simulink model "immd_design_elen_sim2"  (R2013a)
settings: Solver=ode4  StartTime=0.0  StopTime=0.04  FixedStep=Ts  RelTol=1e-3
values from neighbouring files (symbols this model uses):
  Cdc = ma*(Iapeak - Idcc)/(volt_ripple*fsw*2)    [immd_design_elen.m]    (also in immd_efficiency.m = 5e-05; immd_simulation_base.m = 5e-05; sixth_harmonic_report.m = 0.003)
  Lload = Xload/wout_fund    [acemp_sixth.m]    (also in immd_base_varyingmod.m = Xload/wout; immd_design_elen.m = Xload/wout; immd_efficiency.m = Xload/wout; immd_simulation_base.m = Xload/wout)
  ma = 1    [IMMD_design_tool_v01.m]    (also in IMMD_design_tool_v02.m = 0.9; immd_base_varyingmod.m; immd_design_elen.m = 0.8; immd_efficiency.m = 0.85)
  phase = zeros(1,max_number_module)    [immd_base_varyingmod.m]    (also in immd_design_elen.m = [0 90 0 90]; immd_simulation_base.m = zeros(1,n))
  Rin = 10    [immd_design_elen.m]
  Rload = Zload*pf    [acemp_sixth.m]    (also in immd_base_varyingmod.m; immd_design_elen.m; immd_efficiency.m; immd_simulation_base.m)
  Ts = 1e-6    (= 1e-06)    [acemp_sixth.m]    (also in immd_base_varyingmod.m = 1e-05; immd_design_elen.m; immd_efficiency.m; immd_simulation_base.m)
  Vin = Vdc + Rin*(Ptotal/Vdc)    (= 704.609053498)    [immd_design_elen.m]
  wout = 2*pi*fout    (= 314.159265359)    [immd_base_varyingmod.m]    (also in immd_design_elen.m; immd_efficiency.m; immd_simulation_base.m)
undefined symbols (not defined in the file or in its folder): Lin
libraries: powerlib x65, powerlib_meascontrol x30
settings Model: Creator=ugurm  LastModifiedBy=ugurm

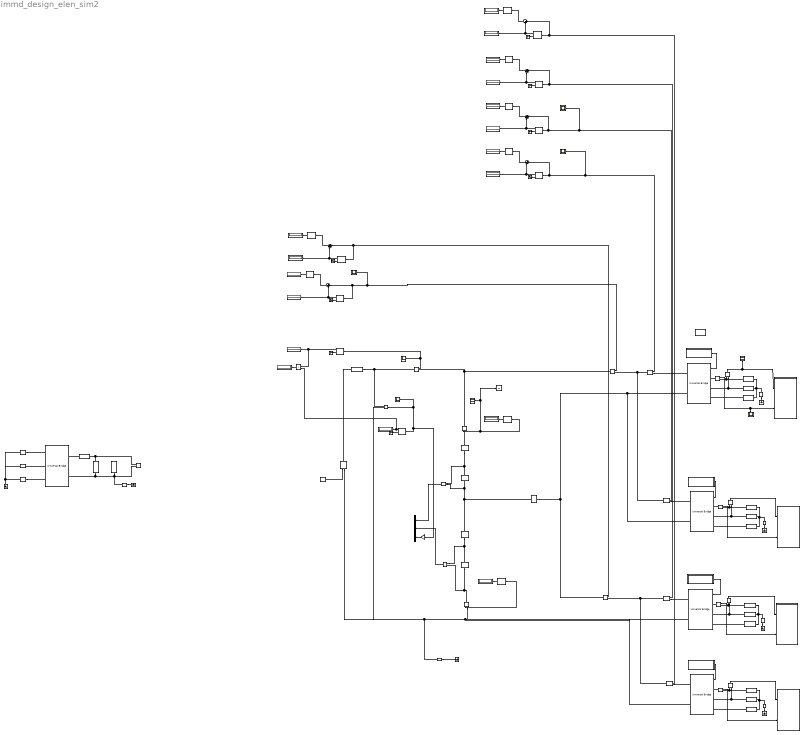
== system immd_design_elen_sim2 ==
  AC Voltage Source : powerlib/Electrical Sources/AC Voltage Source  Amplitude=230*sqrt(2)  Phase=0  Frequency=50  SampleTime=0  Measurements=None
  AC Voltage Source1 : powerlib/Electrical Sources/AC Voltage Source  Amplitude=230*sqrt(2)  Phase=120  Frequency=50  SampleTime=0  Measurements=None
  AC Voltage Source2 : powerlib/Electrical Sources/AC Voltage Source  Amplitude=230*sqrt(2)  Phase=240  Frequency=50  SampleTime=0  Measurements=None
  Constant : Constant  Value=Vin
  Display{1..10,15..21} (17 alike) : Display
  Fourier{1..8} (8 alike) : powerlib_meascontrol/Measurements/Fourier  Freq=fout  n=0  InInit=[20, 0]  Ts=Ts
  Gain : Gain  Gain=0.5
  Gate drive 1 : Subsystem
  Gate drive 2 : Subsystem
  Gate drive 3 : Subsystem
  Gate drive 4 : Subsystem
  Ground{,1..6} (7 alike) : powerlib/Elements/Ground  LConnTagsString=a
  Idc_m{1..13} (13 alike) : powerlib/Measurements/Current Measurement  PhasorSimulation=off  OutputType=Complex  PSBequivalent=0
  Integrator : Integrator
  Mux1 : Mux  Inputs=3
  Product : Product
  RMS1 : powerlib_meascontrol/Measurements/RMS  TrueRMS=on  Freq=50  RMSInit=0  Ts=Ts
  RMS{3..5,10..12} (6 alike) : powerlib_meascontrol/Measurements/RMS  TrueRMS=on  Freq=50  RMSInit=25  Ts=Ts
  RMS2 : powerlib_meascontrol/Measurements/RMS  TrueRMS=on  Freq=100  RMSInit=0  Ts=Ts
  Scope{4,9..10,12..16} (8 alike) : Scope
      Scope10 settings: YMin=-27.5  YMax=27.5  SaveName=ScopeData9
      Scope12 settings: YMin=-15  YMax=17.5  SaveName=Icap
      Scope13 settings: YMin=-15  YMax=17.5  SaveName=Idc1
      Scope14 settings: YMin=-9  SaveName=Iin
      Scope15 settings: YMin=-15  YMax=17.5  SaveName=Idc2
      Scope16 settings: YMin=-15  YMax=17.5  SaveName=Idct
      Scope4 settings: YMin=0  YMax=650  SaveName=Vdcc
      Scope9 settings: YMin=-25  YMax=425  SaveName=ScopeData8
  Series RLC Branch{,1..2,8..10,12..14,16..18} (12 alike) : powerlib/Elements/Series RLC Branch  LConnTagsString=__new0  RConnTagsString=__new0  BranchType=RL  Resistance=Rload  Inductance=Lload  SetiL0=off  InitialCurrent=0  Capacitance=1e-6  Setx0=off  InitialVoltage=0  Measurements=None
  Series RLC Branch{3..4,11,15,19,25} (6 alike) : powerlib/Elements/Series RLC Branch  LConnTagsString=__new0  RConnTagsString=__new0  BranchType=R  Resistance=1e12  Inductance=Lload  SetiL0=off  InitialCurrent=0  Capacitance=1e-6  Setx0=off  InitialVoltage=0  Measurements=None
  Series RLC Branch22 : powerlib/Elements/Series RLC Branch  LConnTagsString=__new0  RConnTagsString=__new0  BranchType=RL  Resistance=1e-3  Inductance=3e-3  SetiL0=off  InitialCurrent=0  Capacitance=1e-6  Setx0=off  InitialVoltage=0  Measurements=None
  Series RLC Branch23 : powerlib/Elements/Series RLC Branch  LConnTagsString=__new0  RConnTagsString=__new0  BranchType=RC  Resistance=1e-3  Inductance=3e-3  SetiL0=off  InitialCurrent=0  Capacitance=5e-3  Setx0=on  InitialVoltage=500  Measurements=None
  Series RLC Branch24 : powerlib/Elements/Series RLC Branch  LConnTagsString=__new0  RConnTagsString=__new0  BranchType=R  Resistance=36.45  Inductance=3e-3  SetiL0=off  InitialCurrent=0  Capacitance=1e-6  Setx0=off  InitialVoltage=0  Measurements=None
  Series RLC Branch26 : powerlib/Elements/Series RLC Branch  LConnTagsString=__new0  RConnTagsString=__new0  BranchType=R  Resistance=Rin  Inductance=Lin  SetiL0=off  InitialCurrent=0  Capacitance=1e-6  Setx0=off  InitialVoltage=0  Measurements=None
  Series RLC Branch27 : powerlib/Elements/Series RLC Branch  LConnTagsString=__new0  RConnTagsString=__new0  BranchType=C  Resistance=100e-6  Inductance=100e-6  SetiL0=off  InitialCurrent=0  Capacitance=Cdc*2  Setx0=off  InitialVoltage=170  Measurements=None
  Series RLC Branch28 : powerlib/Elements/Series RLC Branch  LConnTagsString=__new0  RConnTagsString=__new0  BranchType=R  Resistance=1e-9  Inductance=100e-6  SetiL0=off  InitialCurrent=0  Capacitance=Cdc*2  Setx0=on  InitialVoltage=170  Measurements=None
  Series RLC Branch29 : powerlib/Elements/Series RLC Branch  LConnTagsString=__new0  RConnTagsString=__new0  BranchType=R  Resistance=1e-9  Inductance=100e-6  SetiL0=off  InitialCurrent=0  Capacitance=Cdc*2  Setx0=on  InitialVoltage=170  Measurements=None
  Series RLC Branch30 : powerlib/Elements/Series RLC Branch  LConnTagsString=__new0  RConnTagsString=__new0  BranchType=R  Resistance=1e-9  Inductance=100e-6  SetiL0=off  InitialCurrent=0  Capacitance=Cdc*2  Setx0=on  InitialVoltage=170  Measurements=None
  Series RLC Branch5 : powerlib/Elements/Series RLC Branch  LConnTagsString=__new0  RConnTagsString=__new0  BranchType=C  Resistance=100e-6  Inductance=100e-6  SetiL0=off  InitialCurrent=0  Capacitance=Cdc*2  Setx0=off  InitialVoltage=170  Measurements=None
  Subsystem : Subsystem
  Subsystem1 : Subsystem
  Subsystem2 : Subsystem
  Subsystem3 : Subsystem
  Sum{1..6} (6 alike) : Sum  Inputs=|+-
  Terminator{1..8} (8 alike) : Terminator
  Universal Bridge{,1..3} (4 alike) : powerlib/Power Electronics/Universal Bridge  Arms=3  SnubberResistance=1e5  SnubberCapacitance=inf  Device=IGBT / Diodes  Ron=1e-6  Lon=0  ForwardVoltages="[  0  0  ]"  ForwardVoltage=0  GTOparameters=[ 10e-6 , 20e-6 ]  IGBTparameters=[0,0]  Measurements=None  Measurements_2=None  converterType=Rectifier
  Universal Bridge4 : powerlib/Power Electronics/Universal Bridge  Arms=3  SnubberResistance=1e5  SnubberCapacitance=inf  Device=Diodes  Ron=1e-6  Lon=0  ForwardVoltages="[  0  0  ]"  ForwardVoltage=0  GTOparameters=[ 10e-6 , 20e-6 ]  IGBTparameters=[0,0]  Measurements=None  Measurements_2=None  converterType=Rectifier
  Vdc : powerlib/Electrical Sources/Controlled Voltage Source  Initialize=off  Source_Type=DC  Amplitude=200  Phase=0  Frequency=0  Measurements=None
  Vdc_m{1..4} (4 alike) : powerlib/Measurements/Voltage Measurement  PhasorSimulation=off  OutputType=Complex  PSBequivalent=0
  Voltage Measurement{,1..3} (4 alike) : powerlib/Measurements/Voltage Measurement  PhasorSimulation=off  OutputType=Complex  PSBequivalent=0
  powergui : powerlib/powergui  Priority=1  SimulationMode=Discrete  SolverType=Tustin  SampleTime=Ts  frequency=60  SPID=off  DisableSnubberDevices=off  DisableRonSwitches=off  DisableVfSwitches=off  SwTol=0  Interpol=off  DisplayEquations=off  frequencyindice=0  Pbase=100e6  ErrMax=1e-4  Iterations=50  UnitsV=kV  UnitsW=MW  FunctionMessages=off  echomessages=off  HookPort=off  EnableUseOfTLC=off  x0status=blocks  RestoreLinks=warning  ResistiveCurrentMeasurement=off  Frange=[0:2:500]  Ylog=off  Xlog=on  ShowGrid=off  save=off  variable=ZData  structure=Vdc  ZoomFFT=off  StartTime=0.04  cycles=5  DisplayStyle=5  fundamental=50  FreqAxis=off  MaxFrequency=30000  frequencyindicesteady=1  RmsSteady=1  display=off  Ts=0  methode=off
  wires:
  Gate drive 1/1(gate1) -> Universal Bridge/1
  Vdc_m1/1 -> Scope9/1, Subsystem/1(Vab)
  Idc_m1/1 -> Scope10/1, Subsystem/2(Ia)
  Constant/1 -> Vdc/1
  RMS1/1 -> Display4/1
  Gate drive 2/1(gate1) -> Universal Bridge1/1
  Vdc_m2/1 -> Subsystem1/1(Vab)
  Idc_m2/1 -> Subsystem1/2(Ia)
  Gate drive 3/1(gate1) -> Universal Bridge2/1
  Vdc_m3/1 -> Subsystem2/1(Vab)
  Idc_m3/1 -> Subsystem2/2(Ia)
  Gate drive 4/1(gate1) -> Universal Bridge3/1
  Vdc_m4/1 -> Subsystem3/1(Vab)
  Idc_m4/1 -> Subsystem3/2(Ia)
  Product/1 -> Display3/1
  Fourier3/2 -> Terminator3/1
  Fourier3/1 -> Product/1, Display7/1
  Voltage Measurement1/1 -> Gain/1, Fourier4/1, Scope4/1
  Fourier4/2 -> Terminator5/1
  Fourier4/1 -> Product/2, Display9/1
  Idc_m7/1 -> Scope14/1, Fourier3/1
  RMS2/1 -> Display1/1
  RMS5/1 -> Display6/1
  Sum1/1 -> RMS5/1
  Fourier1/1 -> Sum1/2, Display5/1
  Fourier1/2 -> Terminator1/1
  Idc_m5/1 -> Scope16/1, Fourier1/1, Sum1/1
  RMS4/1 -> Display10/1
  Sum2/1 -> RMS4/1
  Fourier2/1 -> Sum2/2, Display2/1
  Fourier2/2 -> Terminator2/1
  Idc_m10/1 -> Fourier2/1, Sum2/1
  Idc_m11/1 -> Integrator/1, Scope12/1, RMS2/1
  Idc_m9/1 -> RMS1/1
  Voltage Measurement3/1 -> Mux1/2
  Voltage Measurement2/1 -> Mux1/1
  Idc_m8/1 -> Scope13/1, Sum3/1, Fourier5/1
  Idc_m13/1 -> Sum5/1, Fourier7/1
  Idc_m12/1 -> Sum6/1, Fourier8/1
  Idc_m6/1 -> Scope15/1, Sum4/1, Fourier6/1
  RMS3/1 -> Display8/1
  Sum3/1 -> RMS3/1
  Fourier5/1 -> Sum3/2, Display15/1
  Fourier5/2 -> Terminator4/1
  RMS10/1 -> Display16/1
  Sum4/1 -> RMS10/1
  Fourier6/1 -> Sum4/2, Display17/1
  Fourier6/2 -> Terminator6/1
  RMS11/1 -> Display18/1
  Sum5/1 -> RMS11/1
  Fourier7/1 -> Sum5/2, Display19/1
  Fourier7/2 -> Terminator7/1
  RMS12/1 -> Display20/1
  Sum6/1 -> RMS12/1
  Fourier8/1 -> Sum6/2, Display21/1
  Fourier8/2 -> Terminator8/1
  Gain/1 -> Mux1/3
  connections:
  Idc_m1/LConn1 -- Universal Bridge/LConn1
  Series RLC Branch1/LConn1 -- Universal Bridge/LConn2 -- Vdc_m1/LConn2
  Series RLC Branch2/LConn1 -- Universal Bridge/LConn3
  Series RLC Branch/LConn1 -- Idc_m1/RConn1 -- Vdc_m1/LConn1
  Series RLC Branch/RConn1 -- Series RLC Branch4/LConn1 -- Series RLC Branch2/RConn1 -- Series RLC Branch1/RConn1
  Series RLC Branch4/RConn1 -- Ground1/LConn1
  Series RLC Branch3/RConn1 -- Ground/LConn1
  Series RLC Branch5/RConn1 -- Idc_m9/LConn1 -- Voltage Measurement3/LConn2
  Vdc_m2/LConn2 -- Universal Bridge1/LConn2 -- Series RLC Branch9/LConn1
  Vdc_m2/LConn1 -- Series RLC Branch8/LConn1 -- Idc_m2/RConn1
  Series RLC Branch10/RConn1 -- Series RLC Branch8/RConn1 -- Series RLC Branch9/RConn1 -- Series RLC Branch11/LConn1
  Series RLC Branch10/LConn1 -- Universal Bridge1/LConn3
  Idc_m2/LConn1 -- Universal Bridge1/LConn1
  Series RLC Branch11/RConn1 -- Ground2/LConn1
  Vdc_m3/LConn2 -- Universal Bridge2/LConn2 -- Series RLC Branch13/LConn1
  Vdc_m3/LConn1 -- Series RLC Branch12/LConn1 -- Idc_m3/RConn1
  Series RLC Branch14/RConn1 -- Series RLC Branch12/RConn1 -- Series RLC Branch13/RConn1 -- Series RLC Branch15/LConn1
  Series RLC Branch14/LConn1 -- Universal Bridge2/LConn3
  Idc_m3/LConn1 -- Universal Bridge2/LConn1
  Series RLC Branch15/RConn1 -- Ground3/LConn1
  Vdc_m4/LConn2 -- Universal Bridge3/LConn2 -- Series RLC Branch17/LConn1
  Vdc_m4/LConn1 -- Series RLC Branch16/LConn1 -- Idc_m4/RConn1
  Series RLC Branch18/RConn1 -- Series RLC Branch16/RConn1 -- Series RLC Branch17/RConn1 -- Series RLC Branch19/LConn1
  Series RLC Branch18/LConn1 -- Universal Bridge3/LConn3
  Idc_m4/LConn1 -- Universal Bridge3/LConn1
  Series RLC Branch19/RConn1 -- Ground4/LConn1
  Idc_m11/LConn1 -- Idc_m7/RConn1 -- Idc_m5/LConn1
  AC Voltage Source/RConn1 -- Universal Bridge4/LConn1
  Universal Bridge4/LConn2 -- AC Voltage Source1/RConn1
  AC Voltage Source2/RConn1 -- Universal Bridge4/LConn3
  Ground5/LConn1 -- AC Voltage Source/LConn1 -- AC Voltage Source1/LConn1 -- AC Voltage Source2/LConn1
  Series RLC Branch22/RConn1 -- Universal Bridge4/RConn1
  Voltage Measurement/LConn1 -- Series RLC Branch23/LConn1 -- Series RLC Branch22/LConn1
  Series RLC Branch25/RConn1 -- Ground6/LConn1
  Voltage Measurement/LConn2 -- Series RLC Branch24/LConn1 -- Series RLC Branch25/LConn1 -- Series RLC Branch23/RConn1 -- Universal Bridge4/RConn2
  Series RLC Branch26/LConn1 -- Idc_m7/LConn1 -- Voltage Measurement1/LConn1
  Series RLC Branch26/RConn1 -- Vdc/RConn1
  Voltage Measurement2/LConn1 -- Series RLC Branch28/RConn1 -- Series RLC Branch27/LConn1
  Series RLC Branch29/LConn1 -- Voltage Measurement2/LConn2 -- Series RLC Branch27/RConn1 -- Series RLC Branch30/RConn1
  Idc_m6/LConn1 -- Idc_m5/RConn1 -- Idc_m8/LConn1
  Idc_m12/LConn1 -- Idc_m10/RConn1 -- Idc_m13/LConn1
  Series RLC Branch3/LConn1 -- Voltage Measurement1/LConn2 -- Vdc/LConn1 -- Idc_m9/RConn1 -- Universal Bridge1/RConn2 -- Universal Bridge3/RConn2
  Series RLC Branch28/LConn1 -- Idc_m11/RConn1
  Series RLC Branch5/LConn1 -- Series RLC Branch29/RConn1 -- Voltage Measurement3/LConn1
  Universal Bridge/RConn2 -- Universal Bridge2/RConn2 -- Series RLC Branch30/LConn1 -- Idc_m10/LConn1
  Idc_m6/RConn1 -- Universal Bridge/RConn1
  Idc_m8/RConn1 -- Universal Bridge2/RConn1
  Idc_m12/RConn1 -- Universal Bridge1/RConn1
  Idc_m13/RConn1 -- Universal Bridge3/RConn1

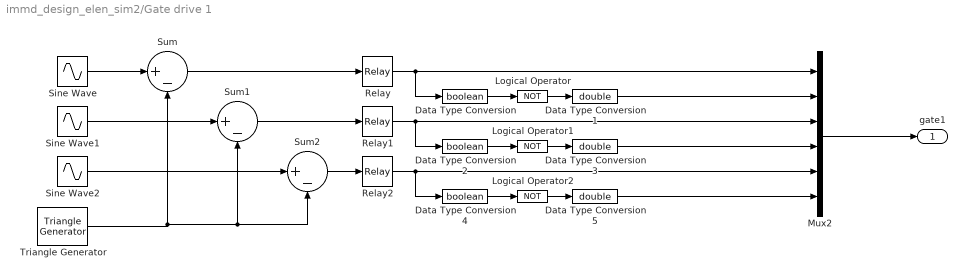
== system immd_design_elen_sim2/Gate drive 1 ==
  Data Type Conversion : DataTypeConversion  OutDataTypeStr=boolean
  Data Type Conversion1 : DataTypeConversion  OutDataTypeStr=double
  Data Type Conversion2 : DataTypeConversion  OutDataTypeStr=boolean
  Data Type Conversion3 : DataTypeConversion  OutDataTypeStr=double
  Data Type Conversion4 : DataTypeConversion  OutDataTypeStr=boolean
  Data Type Conversion5 : DataTypeConversion  OutDataTypeStr=double
  Logical Operator : Logic  Operator=NOT  AllPortsSameDT=off  OutDataTypeStr=boolean
  Logical Operator1 : Logic  Operator=NOT  AllPortsSameDT=off  OutDataTypeStr=boolean
  Logical Operator2 : Logic  Operator=NOT  AllPortsSameDT=off  OutDataTypeStr=boolean
  Mux2 : Mux  Inputs=6
  Relay : Relay
  Relay1 : Relay
  Relay2 : Relay
  Sine Wave : Sin  Amplitude=ma  Frequency=wout  SampleTime=0
  Sine Wave1 : Sin  Amplitude=ma  Frequency=wout  Phase=-2*pi/3  SampleTime=0
  Sine Wave2 : Sin  Amplitude=ma  Frequency=wout  Phase=2*pi/3  SampleTime=0
  Sum : Sum  Inputs=|+-
  Sum1 : Sum  Inputs=|+-
  Sum2 : Sum  Inputs=|+-
  Triangle Generator : powerlib_meascontrol/Pulse & Signal Generators/Triangle Generator  Freq=fsw  Phase=phase(1)  Ts=Ts
  gate1 : Outport
  wires:
  Sine Wave/1 -> Sum/1
  Triangle Generator/1 -> Sum1/2, Sum2/2, Sum/2
  Sine Wave1/1 -> Sum1/1
  Sine Wave2/1 -> Sum2/1
  Sum/1 -> Relay/1
  Sum1/1 -> Relay1/1
  Sum2/1 -> Relay2/1
  Data Type Conversion/1 -> Logical Operator/1
  Relay/1 -> Data Type Conversion/1, Mux2/1
  Logical Operator/1 -> Data Type Conversion1/1
  Data Type Conversion1/1 -> Mux2/2
  Data Type Conversion2/1 -> Logical Operator1/1
  Relay1/1 -> Data Type Conversion2/1, Mux2/3
  Logical Operator1/1 -> Data Type Conversion3/1
  Data Type Conversion3/1 -> Mux2/4
  Data Type Conversion4/1 -> Logical Operator2/1
  Relay2/1 -> Data Type Conversion4/1, Mux2/5
  Logical Operator2/1 -> Data Type Conversion5/1
  Data Type Conversion5/1 -> Mux2/6
  Mux2/1 -> gate1/1

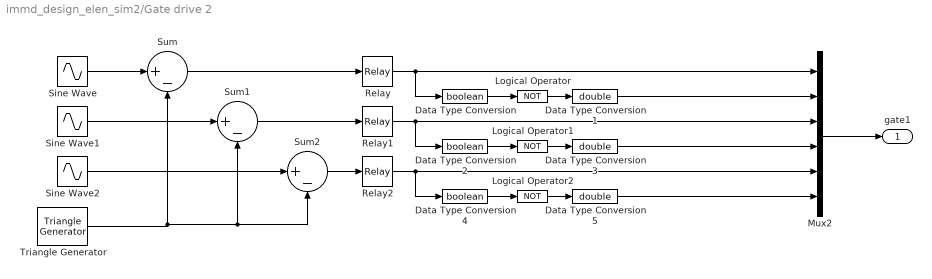
== system immd_design_elen_sim2/Gate drive 2 ==
  Data Type Conversion : DataTypeConversion  OutDataTypeStr=boolean
  Data Type Conversion1 : DataTypeConversion  OutDataTypeStr=double
  Data Type Conversion2 : DataTypeConversion  OutDataTypeStr=boolean
  Data Type Conversion3 : DataTypeConversion  OutDataTypeStr=double
  Data Type Conversion4 : DataTypeConversion  OutDataTypeStr=boolean
  Data Type Conversion5 : DataTypeConversion  OutDataTypeStr=double
  Logical Operator : Logic  Operator=NOT  AllPortsSameDT=off  OutDataTypeStr=boolean
  Logical Operator1 : Logic  Operator=NOT  AllPortsSameDT=off  OutDataTypeStr=boolean
  Logical Operator2 : Logic  Operator=NOT  AllPortsSameDT=off  OutDataTypeStr=boolean
  Mux2 : Mux  Inputs=6
  Relay : Relay
  Relay1 : Relay
  Relay2 : Relay
  Sine Wave : Sin  Amplitude=ma  Frequency=wout  SampleTime=0
  Sine Wave1 : Sin  Amplitude=ma  Frequency=wout  Phase=-2*pi/3  SampleTime=0
  Sine Wave2 : Sin  Amplitude=ma  Frequency=wout  Phase=2*pi/3  SampleTime=0
  Sum : Sum  Inputs=|+-
  Sum1 : Sum  Inputs=|+-
  Sum2 : Sum  Inputs=|+-
  Triangle Generator : powerlib_meascontrol/Pulse & Signal Generators/Triangle Generator  Freq=fsw  Phase=phase(3)  Ts=Ts
  gate1 : Outport
  wires:
  Sine Wave/1 -> Sum/1
  Triangle Generator/1 -> Sum1/2, Sum2/2, Sum/2
  Sine Wave1/1 -> Sum1/1
  Sine Wave2/1 -> Sum2/1
  Sum/1 -> Relay/1
  Sum1/1 -> Relay1/1
  Sum2/1 -> Relay2/1
  Data Type Conversion/1 -> Logical Operator/1
  Relay/1 -> Data Type Conversion/1, Mux2/1
  Logical Operator/1 -> Data Type Conversion1/1
  Data Type Conversion1/1 -> Mux2/2
  Data Type Conversion2/1 -> Logical Operator1/1
  Relay1/1 -> Data Type Conversion2/1, Mux2/3
  Logical Operator1/1 -> Data Type Conversion3/1
  Data Type Conversion3/1 -> Mux2/4
  Data Type Conversion4/1 -> Logical Operator2/1
  Relay2/1 -> Data Type Conversion4/1, Mux2/5
  Logical Operator2/1 -> Data Type Conversion5/1
  Data Type Conversion5/1 -> Mux2/6
  Mux2/1 -> gate1/1

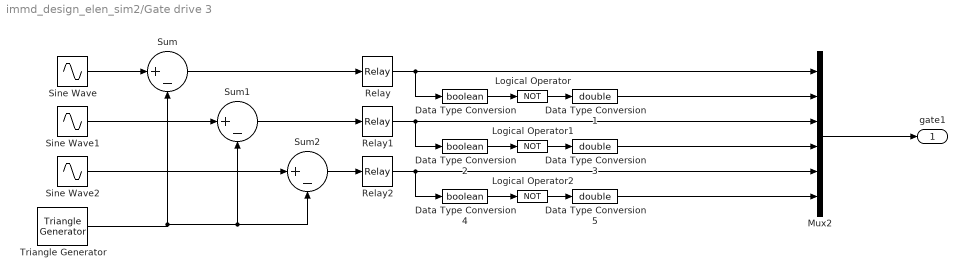
== system immd_design_elen_sim2/Gate drive 3 ==
  Data Type Conversion : DataTypeConversion  OutDataTypeStr=boolean
  Data Type Conversion1 : DataTypeConversion  OutDataTypeStr=double
  Data Type Conversion2 : DataTypeConversion  OutDataTypeStr=boolean
  Data Type Conversion3 : DataTypeConversion  OutDataTypeStr=double
  Data Type Conversion4 : DataTypeConversion  OutDataTypeStr=boolean
  Data Type Conversion5 : DataTypeConversion  OutDataTypeStr=double
  Logical Operator : Logic  Operator=NOT  AllPortsSameDT=off  OutDataTypeStr=boolean
  Logical Operator1 : Logic  Operator=NOT  AllPortsSameDT=off  OutDataTypeStr=boolean
  Logical Operator2 : Logic  Operator=NOT  AllPortsSameDT=off  OutDataTypeStr=boolean
  Mux2 : Mux  Inputs=6
  Relay : Relay
  Relay1 : Relay
  Relay2 : Relay
  Sine Wave : Sin  Amplitude=ma  Frequency=wout  SampleTime=0
  Sine Wave1 : Sin  Amplitude=ma  Frequency=wout  Phase=-2*pi/3  SampleTime=0
  Sine Wave2 : Sin  Amplitude=ma  Frequency=wout  Phase=2*pi/3  SampleTime=0
  Sum : Sum  Inputs=|+-
  Sum1 : Sum  Inputs=|+-
  Sum2 : Sum  Inputs=|+-
  Triangle Generator : powerlib_meascontrol/Pulse & Signal Generators/Triangle Generator  Freq=fsw  Phase=phase(2)  Ts=Ts
  gate1 : Outport
  wires:
  Sine Wave/1 -> Sum/1
  Triangle Generator/1 -> Sum1/2, Sum2/2, Sum/2
  Sine Wave1/1 -> Sum1/1
  Sine Wave2/1 -> Sum2/1
  Sum/1 -> Relay/1
  Sum1/1 -> Relay1/1
  Sum2/1 -> Relay2/1
  Data Type Conversion/1 -> Logical Operator/1
  Relay/1 -> Data Type Conversion/1, Mux2/1
  Logical Operator/1 -> Data Type Conversion1/1
  Data Type Conversion1/1 -> Mux2/2
  Data Type Conversion2/1 -> Logical Operator1/1
  Relay1/1 -> Data Type Conversion2/1, Mux2/3
  Logical Operator1/1 -> Data Type Conversion3/1
  Data Type Conversion3/1 -> Mux2/4
  Data Type Conversion4/1 -> Logical Operator2/1
  Relay2/1 -> Data Type Conversion4/1, Mux2/5
  Logical Operator2/1 -> Data Type Conversion5/1
  Data Type Conversion5/1 -> Mux2/6
  Mux2/1 -> gate1/1

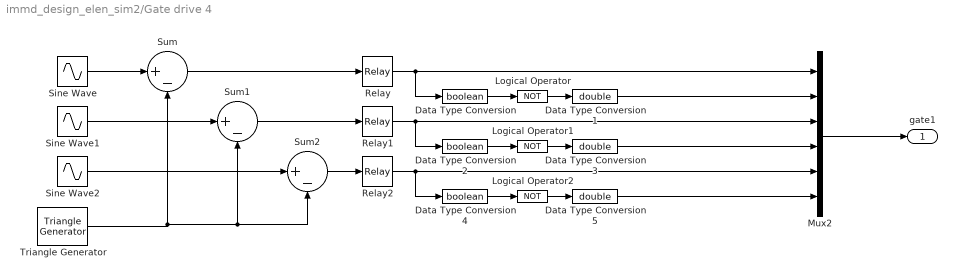
== system immd_design_elen_sim2/Gate drive 4 ==
  Data Type Conversion : DataTypeConversion  OutDataTypeStr=boolean
  Data Type Conversion1 : DataTypeConversion  OutDataTypeStr=double
  Data Type Conversion2 : DataTypeConversion  OutDataTypeStr=boolean
  Data Type Conversion3 : DataTypeConversion  OutDataTypeStr=double
  Data Type Conversion4 : DataTypeConversion  OutDataTypeStr=boolean
  Data Type Conversion5 : DataTypeConversion  OutDataTypeStr=double
  Logical Operator : Logic  Operator=NOT  AllPortsSameDT=off  OutDataTypeStr=boolean
  Logical Operator1 : Logic  Operator=NOT  AllPortsSameDT=off  OutDataTypeStr=boolean
  Logical Operator2 : Logic  Operator=NOT  AllPortsSameDT=off  OutDataTypeStr=boolean
  Mux2 : Mux  Inputs=6
  Relay : Relay
  Relay1 : Relay
  Relay2 : Relay
  Sine Wave : Sin  Amplitude=ma  Frequency=wout  SampleTime=0
  Sine Wave1 : Sin  Amplitude=ma  Frequency=wout  Phase=-2*pi/3  SampleTime=0
  Sine Wave2 : Sin  Amplitude=ma  Frequency=wout  Phase=2*pi/3  SampleTime=0
  Sum : Sum  Inputs=|+-
  Sum1 : Sum  Inputs=|+-
  Sum2 : Sum  Inputs=|+-
  Triangle Generator : powerlib_meascontrol/Pulse & Signal Generators/Triangle Generator  Freq=fsw  Phase=phase(4)  Ts=Ts
  gate1 : Outport
  wires:
  Sine Wave/1 -> Sum/1
  Triangle Generator/1 -> Sum1/2, Sum2/2, Sum/2
  Sine Wave1/1 -> Sum1/1
  Sine Wave2/1 -> Sum2/1
  Sum/1 -> Relay/1
  Sum1/1 -> Relay1/1
  Sum2/1 -> Relay2/1
  Data Type Conversion/1 -> Logical Operator/1
  Relay/1 -> Data Type Conversion/1, Mux2/1
  Logical Operator/1 -> Data Type Conversion1/1
  Data Type Conversion1/1 -> Mux2/2
  Data Type Conversion2/1 -> Logical Operator1/1
  Relay1/1 -> Data Type Conversion2/1, Mux2/3
  Logical Operator1/1 -> Data Type Conversion3/1
  Data Type Conversion3/1 -> Mux2/4
  Data Type Conversion4/1 -> Logical Operator2/1
  Relay2/1 -> Data Type Conversion4/1, Mux2/5
  Logical Operator2/1 -> Data Type Conversion5/1
  Data Type Conversion5/1 -> Mux2/6
  Mux2/1 -> gate1/1

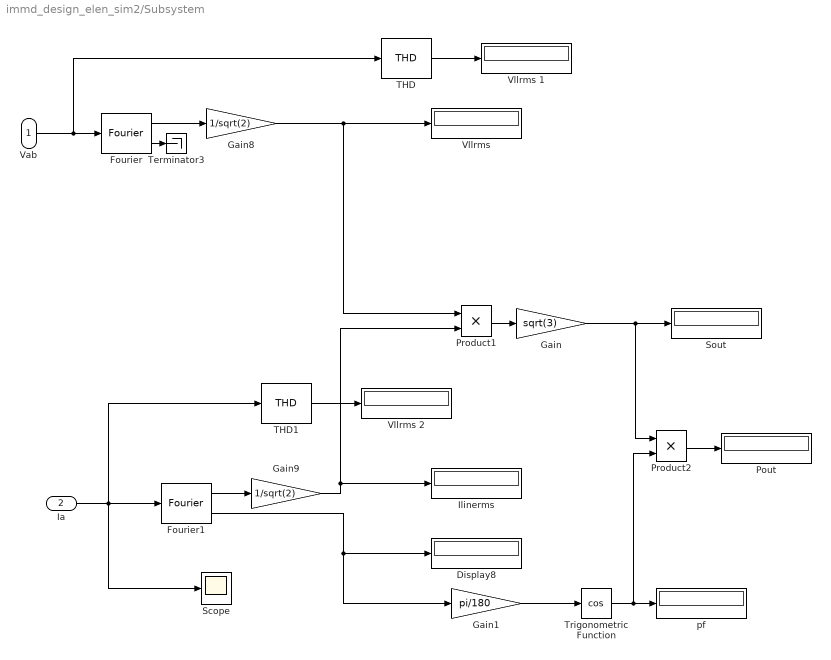
== system immd_design_elen_sim2/Subsystem ==
  Vab : Inport
  Ia : Inport  Port=2
  Display8 : Display
  Fourier : powerlib_meascontrol/Measurements/Fourier  Freq=fout  n=1  InInit=[0, 0]  Ts=Ts
  Fourier1 : powerlib_meascontrol/Measurements/Fourier  Freq=fout  n=1  InInit=[0, 0]  Ts=Ts
  Gain : Gain  Gain=sqrt(3)
  Gain1 : Gain  Gain=pi/180
  Gain8 : Gain  Gain=1/sqrt(2)
  Gain9 : Gain  Gain=1/sqrt(2)
  "Ilinerms " : Display
  Pout : Display
  Product1 : Product
  Product2 : Product
  Scope : Scope
      settings: YMin=-10  YMax=10  SaveName=ScopeData4
  Sout : Display
      settings: Format=short_e
  THD : powerlib_meascontrol/Measurements/THD  Freq=fout  Ts=0
  THD1 : powerlib_meascontrol/Measurements/THD  Freq=fout  Ts=0
  Terminator3 : Terminator
  Trigonometric Function : Trigonometry  Operator=cos
  "Vllrms " : Display
  Vllrms 1 : Display
  Vllrms 2 : Display
  pf : Display
  wires:
  Gain8/1 -> Product1/1, "Vllrms "/1
  Gain9/1 -> "Ilinerms "/1, Product1/2
  Ia/1 -> THD1/1, Scope/1, Fourier1/1
  Fourier1/1 -> Gain9/1
  Vab/1 -> THD/1, Fourier/1
  Fourier/1 -> Gain8/1
  Product1/1 -> Gain/1
  Gain/1 -> Product2/1, Sout/1
  Fourier1/2 -> Gain1/1, Display8/1
  Trigonometric Function/1 -> Product2/2, pf/1
  Gain1/1 -> Trigonometric Function/1
  Product2/1 -> Pout/1
  Fourier/2 -> Terminator3/1
  THD/1 -> Vllrms 1/1
  THD1/1 -> Vllrms 2/1

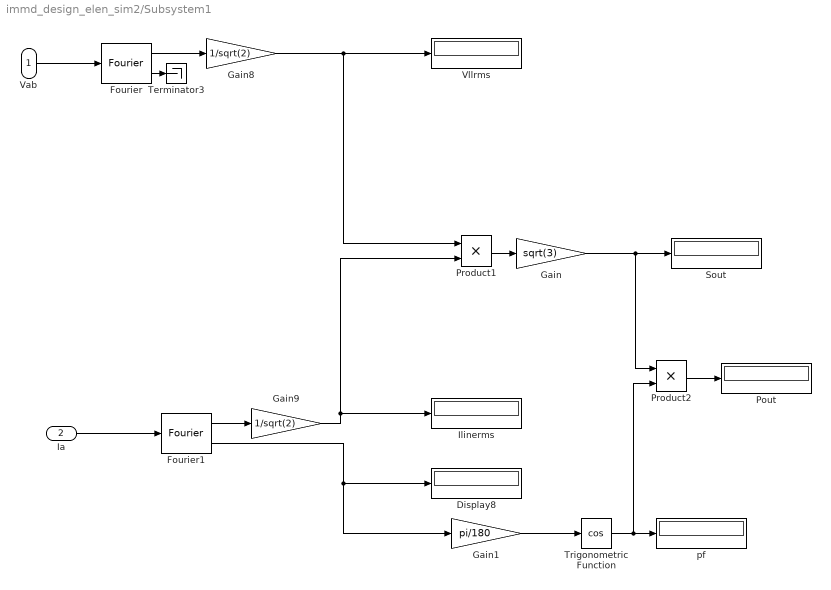
== system immd_design_elen_sim2/Subsystem1 ==
  Vab : Inport
  Ia : Inport  Port=2
  Display8 : Display
  Fourier : powerlib_meascontrol/Measurements/Fourier  Freq=fout  n=1  InInit=[0, 0]  Ts=Ts
  Fourier1 : powerlib_meascontrol/Measurements/Fourier  Freq=fout  n=1  InInit=[0, 0]  Ts=Ts
  Gain : Gain  Gain=sqrt(3)
  Gain1 : Gain  Gain=pi/180
  Gain8 : Gain  Gain=1/sqrt(2)
  Gain9 : Gain  Gain=1/sqrt(2)
  "Ilinerms " : Display
  Pout : Display
  Product1 : Product
  Product2 : Product
  Sout : Display
      settings: Format=short_e
  Terminator3 : Terminator
  Trigonometric Function : Trigonometry  Operator=cos
  "Vllrms " : Display
  pf : Display
  wires:
  Gain8/1 -> Product1/1, "Vllrms "/1
  Gain9/1 -> "Ilinerms "/1, Product1/2
  Ia/1 -> Fourier1/1
  Fourier1/1 -> Gain9/1
  Vab/1 -> Fourier/1
  Fourier/1 -> Gain8/1
  Product1/1 -> Gain/1
  Gain/1 -> Product2/1, Sout/1
  Fourier1/2 -> Gain1/1, Display8/1
  Trigonometric Function/1 -> Product2/2, pf/1
  Gain1/1 -> Trigonometric Function/1
  Product2/1 -> Pout/1
  Fourier/2 -> Terminator3/1

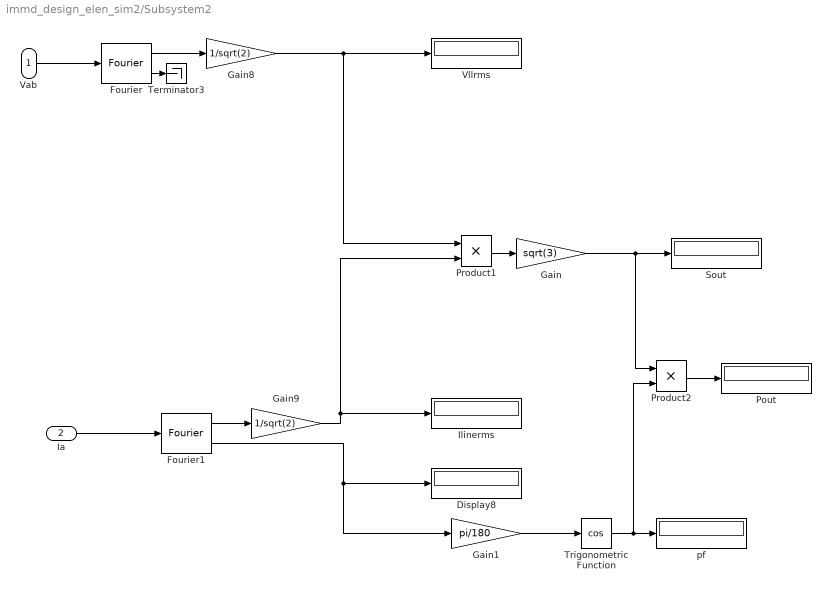
== system immd_design_elen_sim2/Subsystem2 ==
  Vab : Inport
  Ia : Inport  Port=2
  Display8 : Display
  Fourier : powerlib_meascontrol/Measurements/Fourier  Freq=fout  n=1  InInit=[0, 0]  Ts=Ts
  Fourier1 : powerlib_meascontrol/Measurements/Fourier  Freq=fout  n=1  InInit=[0, 0]  Ts=Ts
  Gain : Gain  Gain=sqrt(3)
  Gain1 : Gain  Gain=pi/180
  Gain8 : Gain  Gain=1/sqrt(2)
  Gain9 : Gain  Gain=1/sqrt(2)
  "Ilinerms " : Display
  Pout : Display
  Product1 : Product
  Product2 : Product
  Sout : Display
      settings: Format=short_e
  Terminator3 : Terminator
  Trigonometric Function : Trigonometry  Operator=cos
  "Vllrms " : Display
  pf : Display
  wires:
  Gain8/1 -> Product1/1, "Vllrms "/1
  Gain9/1 -> "Ilinerms "/1, Product1/2
  Ia/1 -> Fourier1/1
  Fourier1/1 -> Gain9/1
  Vab/1 -> Fourier/1
  Fourier/1 -> Gain8/1
  Product1/1 -> Gain/1
  Gain/1 -> Product2/1, Sout/1
  Fourier1/2 -> Gain1/1, Display8/1
  Trigonometric Function/1 -> Product2/2, pf/1
  Gain1/1 -> Trigonometric Function/1
  Product2/1 -> Pout/1
  Fourier/2 -> Terminator3/1

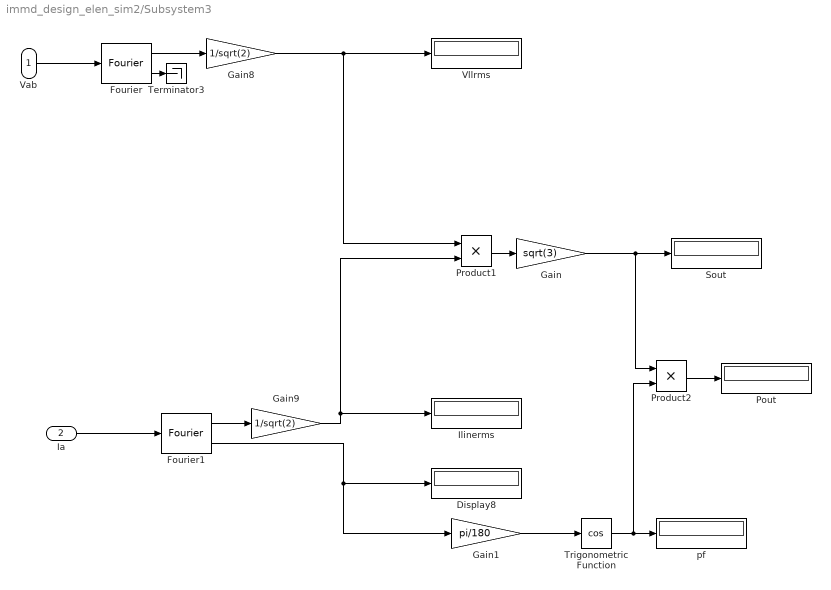
== system immd_design_elen_sim2/Subsystem3 ==
  Vab : Inport
  Ia : Inport  Port=2
  Display8 : Display
  Fourier : powerlib_meascontrol/Measurements/Fourier  Freq=fout  n=1  InInit=[0, 0]  Ts=Ts
  Fourier1 : powerlib_meascontrol/Measurements/Fourier  Freq=fout  n=1  InInit=[0, 0]  Ts=Ts
  Gain : Gain  Gain=sqrt(3)
  Gain1 : Gain  Gain=pi/180
  Gain8 : Gain  Gain=1/sqrt(2)
  Gain9 : Gain  Gain=1/sqrt(2)
  "Ilinerms " : Display
  Pout : Display
  Product1 : Product
  Product2 : Product
  Sout : Display
      settings: Format=short_e
  Terminator3 : Terminator
  Trigonometric Function : Trigonometry  Operator=cos
  "Vllrms " : Display
  pf : Display
  wires:
  Gain8/1 -> Product1/1, "Vllrms "/1
  Gain9/1 -> "Ilinerms "/1, Product1/2
  Ia/1 -> Fourier1/1
  Fourier1/1 -> Gain9/1
  Vab/1 -> Fourier/1
  Fourier/1 -> Gain8/1
  Product1/1 -> Gain/1
  Gain/1 -> Product2/1, Sout/1
  Fourier1/2 -> Gain1/1, Display8/1
  Trigonometric Function/1 -> Product2/2, pf/1
  Gain1/1 -> Trigonometric Function/1
  Product2/1 -> Pout/1
  Fourier/2 -> Terminator3/1
